simulink model "StabilityControllerSpeed"  (R2022b)
settings: configuration reference "WheelSimConfiguration2016" (kept outside this file)
undefined symbols (not defined in the file): simulator
settings Model: Creator=At  LastModifiedBy=ateay
settings ConfigSetRef: SourceName=WheelSimConfiguration2016  SourceLocation=Base Workspace

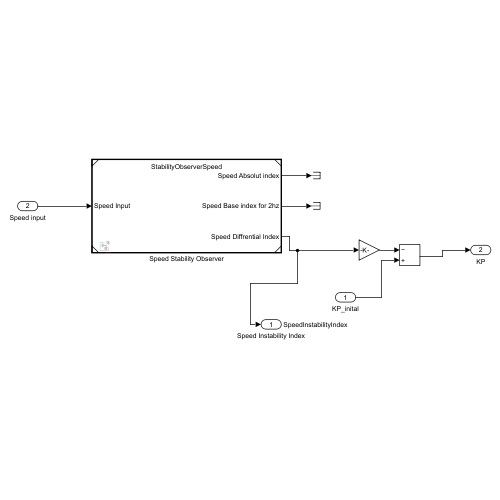
[thumbnail: Simulink's stored preview of the top-level diagram]
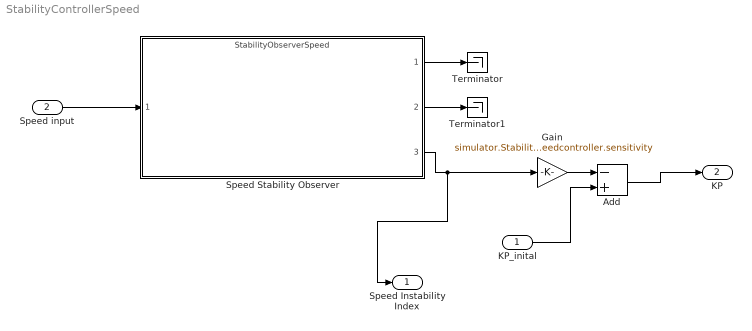
== system StabilityControllerSpeed ==
  KP_inital : Inport
  "Speed input " : Inport  Port=2
  Add : Sum  Inputs=-+
  Gain : Gain  Gain=simulator.Stabilityspeedcontroller.sensitivity
  Speed Stability Observer : ModelReference  ModelNameDialog=StabilityObserverSpeed.slx  SimulationMode=Normal  ModelReferenceVersion=1.23
  Terminator : Terminator
  Terminator1 : Terminator
  Speed Instability Index : Outport  SignalName=SpeedInstabilityIndex
  KP : Outport  Port=2
  wires:
  "Speed input "/1 -> Speed Stability Observer/1
  Speed Stability Observer/1 -> Terminator/1
  Speed Stability Observer/2 -> Terminator1/1
  KP_inital/1 -> Add/2
  Gain/1 -> Add/1
  Add/1 -> KP/1
  Speed Stability Observer/3 -> Speed Instability Index/1, Gain/1
